simulink model "bloques_PMSM_v2"  (R2020b)
settings: Solver=VariableStepAuto  StartTime=0.0  StopTime=10.0  RelTol=1e-3
settings Model: Creator=JJVS  LastModifiedBy=jacob

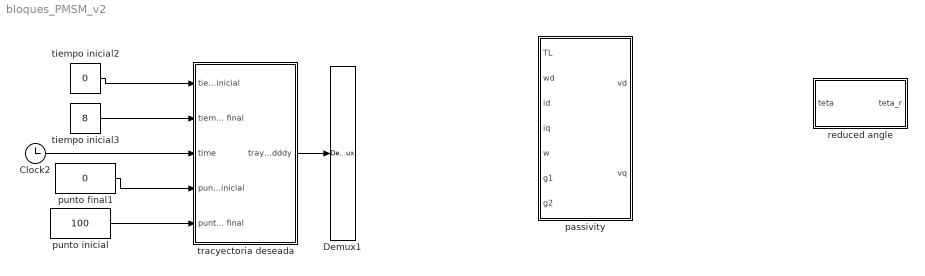
== system bloques_PMSM_v2 ==
  Clock2 : Clock
  Demux1 : Demux  Outputs=5
      settings: DisplayOption=none
  passivity : MATLAB Function  TreatAsAtomicUnit=on
  punto final1 : Constant  Value=0
  punto inicial : Constant  Value=100
  reduced angle : MATLAB Function  TreatAsAtomicUnit=on
  tiempo inicial2 : Constant  Value=0
  tiempo inicial3 : Constant  Value=8
  tracyectoria deseada : Subsystem
  wires:
  tiempo inicial2/1 -> tracyectoria deseada/1(tiempo inicial)
  tiempo inicial3/1 -> tracyectoria deseada/2(tiempo final)
  tracyectoria deseada/1(trayectoria y - ddddy) -> Demux1/1
  Clock2/1 -> tracyectoria deseada/3(time)
  punto inicial/1 -> tracyectoria deseada/5(punto final)
  punto final1/1 -> tracyectoria deseada/4(punto inicial)

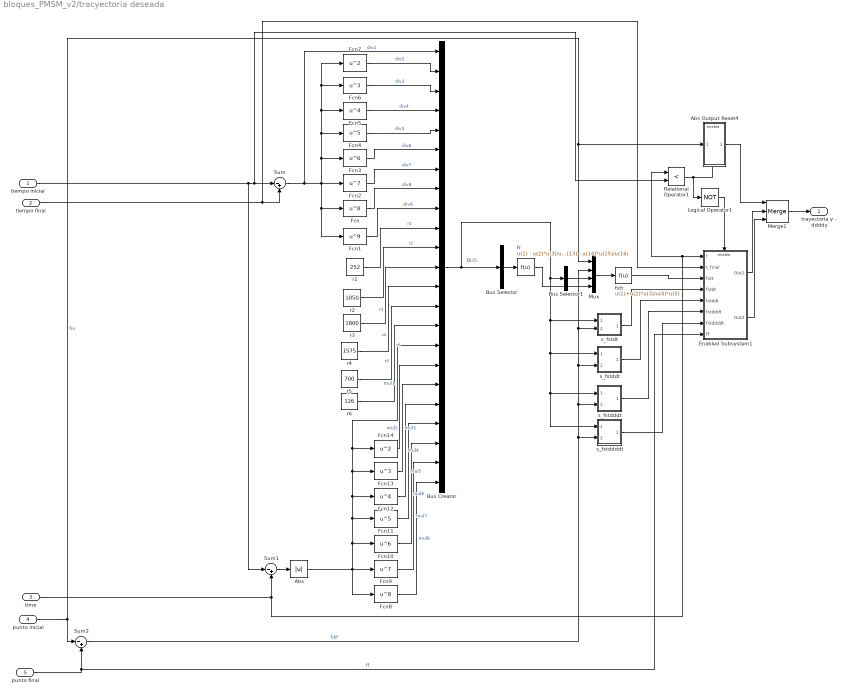
== system bloques_PMSM_v2/tracyectoria deseada ==
  note: BUS
  tiempo inicial : Inport
  tiempo final : Inport  Port=2
  time : Inport  Port=3
  punto inicial : Inport  Port=4
  punto final : Inport  Port=5
  Abs : Abs  SaturateOnIntegerOverflow=on
  Abs Output Reset4 : Subsystem  TreatAsAtomicUnit=on
  Bus Creator : BusCreator  Inputs=23
  Bus Selector : BusSelector  OutputSignals=r1,r2,mul1,div1,r3,mul2,div2,r4,mul3,div3,r5,mul4,div4,r6,mul5,div5  OutputAsBus=on
  Bus Selector1 : BusSelector  OutputSignals=mul5,div5  OutputAsBus=on
  Enabled Subsystem1 : Subsystem  TreatAsAtomicUnit=on
  Fcn : Fcn  Expr=u^8
  Fcn1 : Fcn  Expr=u^9
  Fcn10 : Fcn  Expr=u^6
  Fcn11 : Fcn  Expr=u^5
  Fcn12 : Fcn  Expr=u^4
  Fcn13 : Fcn  Expr=u^3
  Fcn14 : Fcn  Expr=u^2
  Fcn2 : Fcn  Expr=u^7
  Fcn3 : Fcn  Expr=u^6
  Fcn4 : Fcn  Expr=u^5
  Fcn5 : Fcn  Expr=u^4
  Fcn6 : Fcn  Expr=u^3
  Fcn7 : Fcn  Expr=u^2
  Fcn8 : Fcn  Expr=u^8
  Fcn9 : Fcn  Expr=u^7
  Logical Operator1 : Logic  Operator=NOT  AllPortsSameDT=off
  Merge1 : Merge  Inputs=3
  Mux : Mux
  Relational Operator1 : RelationalOperator  Operator=<  RndMeth=Nearest
  Sum : Sum  Inputs=|-+  SaturateOnIntegerOverflow=on
  Sum1 : Sum  Inputs=|-+  SaturateOnIntegerOverflow=on
  Sum2 : Sum  Inputs=|-+  SaturateOnIntegerOverflow=on
  fr : Fcn  Expr=u(1) - u(2)*u(3)/u(4)+u(5)*u(6)/u(7) - u(8)*u(9)/u(10) + u(11)*u(12)/u(13) - u(14)*u(15)/u(16)
  fstt : Fcn  Expr=u(1)+u(2)*u(3)/u(4)*u(5)
  r1 : Constant  Value=252
  r2 : Constant  Value=1050
  r3 : Constant  Value=1800
  r4 : Constant  Value=1575
  r5 : Constant  Value=700
  r6 : Constant  Value=126
  s_fstddddt : Subsystem
  s_fstdddt : Subsystem
  s_fstddt : Subsystem
  s_fstdt : Subsystem
  trayectoria y - ddddy : Outport  VectorParamsAs1DForOutWhenUnconnected=off
  wires:
  punto inicial/1 -> Mux/1, Abs Output Reset4/1(In1), Sum2/1  "fin"
  Bus Selector/1 -> fr/1
  Bus Selector1/1 -> Mux/3
  fr/1 -> Mux/4
  Mux/1 -> fstt/1
  punto final/1 -> Sum2/2, Enabled Subsystem1/8(ff)  "ff"
  tiempo inicial/1 -> Sum1/1, Sum/1, Relational Operator1/2
  Sum1/1 -> Abs/1
  Sum/1 -> Fcn2/1, Fcn3/1, Fcn4/1, Fcn5/1, Fcn6/1, Fcn7/1, Fcn/1, Fcn1/1, Bus Creator/1  "div1"
  Abs/1 -> Fcn13/1, Fcn14/1, Bus Creator/16, Fcn12/1, Fcn11/1, Fcn10/1, Fcn9/1, Fcn8/1  "mul1"
  Fcn7/1 -> Bus Creator/2  "div2"
  Fcn6/1 -> Bus Creator/3  "div3"
  Fcn5/1 -> Bus Creator/4  "div4"
  Fcn4/1 -> Bus Creator/5  "div5"
  Fcn3/1 -> Bus Creator/6  "div6"
  Fcn/1 -> Bus Creator/8  "div8"
  Fcn2/1 -> Bus Creator/7  "div7"
  Fcn1/1 -> Bus Creator/9  "div9"
  r1/1 -> Bus Creator/10  "r1"
  r2/1 -> Bus Creator/11  "r2"
  r3/1 -> Bus Creator/12  "r3"
  r4/1 -> Bus Creator/13  "r4"
  r5/1 -> Bus Creator/14  "r5"
  r6/1 -> Bus Creator/15  "r6"
  Fcn14/1 -> Bus Creator/17  "mul2"
  Fcn13/1 -> Bus Creator/18  "mul3"
  Fcn12/1 -> Bus Creator/19  "mul4"
  Fcn11/1 -> Bus Creator/20  "mul5"
  Fcn10/1 -> Bus Creator/21  "mul6"
  Fcn9/1 -> Bus Creator/22  "mul7"
  Fcn8/1 -> Bus Creator/23  "mul8"
  tiempo final/1 -> Sum/2, Enabled Subsystem1/2(t_final)
  time/1 -> Sum1/2, Enabled Subsystem1/1(t), Relational Operator1/1
  Merge1/1 -> trayectoria y - ddddy/1
  Bus Creator/1 -> Bus Selector1/1, s_fstdt/1(In1), s_fstddt/1(In1), s_fstdddt/1(In1), s_fstddddt/1(In1), Bus Selector/1
  Sum2/1 -> Mux/2, s_fstdt/2(In2), s_fstddt/2(In2), s_fstdddt/2(In2), s_fstddddt/2(In2)  "fdif"
  Relational Operator1/1 -> Abs Output Reset4/Enable, Logical Operator1/1
  Logical Operator1/1 -> Enabled Subsystem1/Enable
  Enabled Subsystem1/1(Out1) -> Merge1/2
  Abs Output Reset4/1(Out) -> Merge1/1
  fstt/1 -> Enabled Subsystem1/3(fstt)
  s_fstdt/1(fstdt) -> Enabled Subsystem1/4(fstdt)
  s_fstddt/1(fstddt) -> Enabled Subsystem1/5(fstddt)
  s_fstdddt/1(fstdddt) -> Enabled Subsystem1/6(fstdddt)
  s_fstddddt/1(fstddddt) -> Enabled Subsystem1/7(fstddddt)
  Enabled Subsystem1/2(Out2) -> Merge1/3

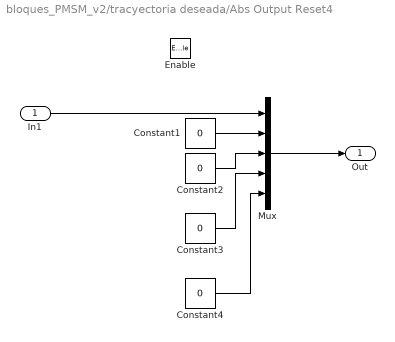
== system bloques_PMSM_v2/tracyectoria deseada/Abs Output Reset4 ==
  In1 : Inport  PortDimensions=1
  Enable : EnablePort
  Constant{1..4} (4 alike) : Constant  Value=0
  Mux : Mux  Inputs=5
  Out : Outport  InitialOutput=0  VectorParamsAs1DForOutWhenUnconnected=off
  wires:
  Mux/1 -> Out/1
  In1/1 -> Mux/1
  Constant1/1 -> Mux/2
  Constant2/1 -> Mux/3
  Constant3/1 -> Mux/4
  Constant4/1 -> Mux/5

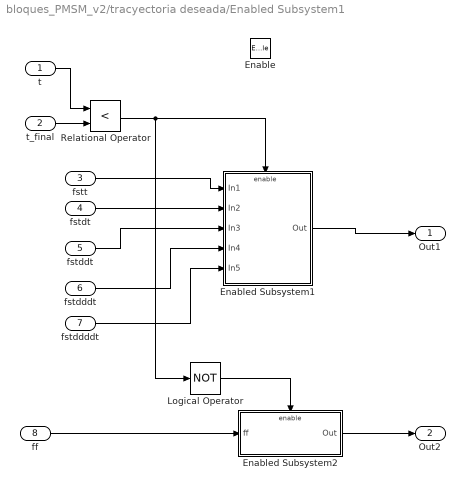
== system bloques_PMSM_v2/tracyectoria deseada/Enabled Subsystem1 ==
  t : Inport  PortDimensions=1
  t_final : Inport  Port=2  PortDimensions=1
  fstt : Inport  Port=3  PortDimensions=1
  fstdt : Inport  Port=4  PortDimensions=1
  fstddt : Inport  Port=5  PortDimensions=1
  fstdddt : Inport  Port=6  PortDimensions=1
  fstddddt : Inport  Port=7  PortDimensions=1
  ff : Inport  Port=8  PortDimensions=1
  Enable : EnablePort
  Enabled Subsystem1 : Subsystem  TreatAsAtomicUnit=on
  Enabled Subsystem2 : Subsystem  TreatAsAtomicUnit=on
  Logical Operator : Logic  Operator=NOT  AllPortsSameDT=off
  Relational Operator : RelationalOperator  Operator=<  RndMeth=Nearest
  Out1 : Outport  VectorParamsAs1DForOutWhenUnconnected=off
  Out2 : Outport  Port=2  VectorParamsAs1DForOutWhenUnconnected=off
  wires:
  Logical Operator/1 -> Enabled Subsystem2/Enable
  Relational Operator/1 -> Logical Operator/1, Enabled Subsystem1/Enable
  t/1 -> Relational Operator/1
  ff/1 -> Enabled Subsystem2/1(ff)
  fstt/1 -> Enabled Subsystem1/1(In1)
  fstdt/1 -> Enabled Subsystem1/2(In2)
  fstddt/1 -> Enabled Subsystem1/3(In3)
  fstdddt/1 -> Enabled Subsystem1/4(In4)
  fstddddt/1 -> Enabled Subsystem1/5(In5)
  t_final/1 -> Relational Operator/2
  Enabled Subsystem1/1(Out) -> Out1/1
  Enabled Subsystem2/1(Out) -> Out2/1

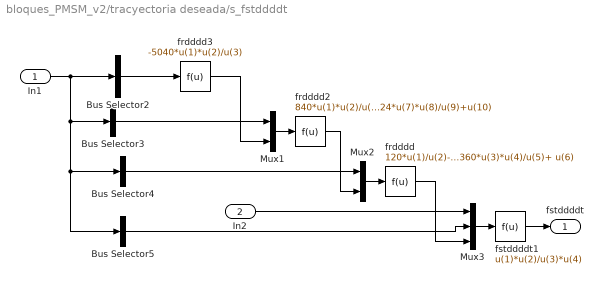
== system bloques_PMSM_v2/tracyectoria deseada/s_fstddddt ==
  In1 : Inport  PortDimensions=23
  In2 : Inport  Port=2  PortDimensions=1
  Bus Selector2 : BusSelector  OutputSignals=r6,mul5,div9  OutputAsBus=on
  Bus Selector3 : BusSelector  OutputSignals=r3,mul2,div6,r4,mul3,div7,r5,mul4,div8  OutputAsBus=on
  Bus Selector4 : BusSelector  OutputSignals=r1,div4,r2,mul1,div5  OutputAsBus=on
  Bus Selector5 : BusSelector  OutputSignals=mul1,div1  OutputAsBus=on
  Mux1 : Mux  Inputs=2
  Mux2 : Mux  Inputs=2
  Mux3 : Mux  Inputs=3
  frdddd : Fcn  Expr=120*u(1)/u(2)-360*u(3)*u(4)/u(5)+ u(6)
  frdddd2 : Fcn  Expr=840*u(1)*u(2)/u(3)-1680*u(4)*u(5)/u(6)+3024*u(7)*u(8)/u(9)+u(10)
  frdddd3 : Fcn  Expr=-5040*u(1)*u(2)/u(3)
  fstddddt1 : Fcn  Expr=u(1)*u(2)/u(3)*u(4)
  fstddddt : Outport  VectorParamsAs1DForOutWhenUnconnected=off
  wires:
  Bus Selector2/1 -> frdddd3/1
  Mux1/1 -> frdddd2/1
  frdddd3/1 -> Mux1/2
  Bus Selector3/1 -> Mux1/1
  Mux2/1 -> frdddd/1
  frdddd2/1 -> Mux2/2
  Bus Selector4/1 -> Mux2/1
  Mux3/1 -> fstddddt1/1
  frdddd/1 -> Mux3/3
  Bus Selector5/1 -> Mux3/2
  In1/1 -> Bus Selector2/1, Bus Selector3/1, Bus Selector4/1, Bus Selector5/1
  In2/1 -> Mux3/1
  fstddddt1/1 -> fstddddt/1

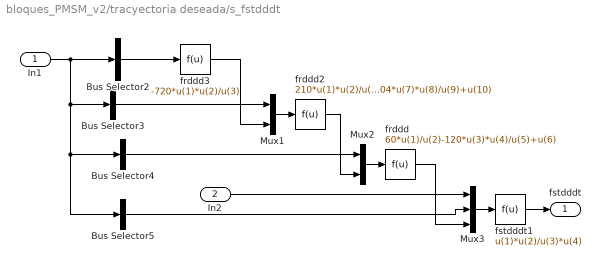
== system bloques_PMSM_v2/tracyectoria deseada/s_fstdddt ==
  In1 : Inport  PortDimensions=23
  In2 : Inport  Port=2  PortDimensions=1
  Bus Selector2 : BusSelector  OutputSignals=r6,mul5,div8  OutputAsBus=on
  Bus Selector3 : BusSelector  OutputSignals=r3,mul2,div5,r4,mul3,div6,r5,mul4,div7  OutputAsBus=on
  Bus Selector4 : BusSelector  OutputSignals=r1,div3,r2,mul1,div4  OutputAsBus=on
  Bus Selector5 : BusSelector  OutputSignals=mul2,div2  OutputAsBus=on
  Mux1 : Mux  Inputs=2
  Mux2 : Mux  Inputs=2
  Mux3 : Mux  Inputs=3
  frddd : Fcn  Expr=60*u(1)/u(2)-120*u(3)*u(4)/u(5)+u(6)
  frddd2 : Fcn  Expr=210*u(1)*u(2)/u(3)-336*u(4)*u(5)/u(6)+504*u(7)*u(8)/u(9)+u(10)
  frddd3 : Fcn  Expr=-720*u(1)*u(2)/u(3)
  fstdddt1 : Fcn  Expr=u(1)*u(2)/u(3)*u(4)
  fstdddt : Outport  VectorParamsAs1DForOutWhenUnconnected=off
  wires:
  fstdddt1/1 -> fstdddt/1
  In2/1 -> Mux3/1
  In1/1 -> Bus Selector5/1, Bus Selector4/1, Bus Selector3/1, Bus Selector2/1
  Bus Selector5/1 -> Mux3/2
  frddd/1 -> Mux3/3
  Mux3/1 -> fstdddt1/1
  Bus Selector4/1 -> Mux2/1
  frddd2/1 -> Mux2/2
  Mux2/1 -> frddd/1
  Bus Selector3/1 -> Mux1/1
  frddd3/1 -> Mux1/2
  Mux1/1 -> frddd2/1
  Bus Selector2/1 -> frddd3/1

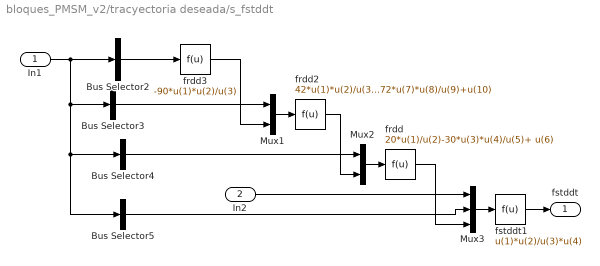
== system bloques_PMSM_v2/tracyectoria deseada/s_fstddt ==
  In1 : Inport  PortDimensions=23
  In2 : Inport  Port=2  PortDimensions=1
  Bus Selector2 : BusSelector  OutputSignals=r6,mul5,div7  OutputAsBus=on
  Bus Selector3 : BusSelector  OutputSignals=r3,mul2,div4,r4,mul3,div5,r5,mul4,div6  OutputAsBus=on
  Bus Selector4 : BusSelector  OutputSignals=r1,div2,r2,mul1,div3  OutputAsBus=on
  Bus Selector5 : BusSelector  OutputSignals=mul3,div3  OutputAsBus=on
  Mux1 : Mux  Inputs=2
  Mux2 : Mux  Inputs=2
  Mux3 : Mux  Inputs=3
  frdd : Fcn  Expr=20*u(1)/u(2)-30*u(3)*u(4)/u(5)+ u(6)
  frdd2 : Fcn  Expr=42*u(1)*u(2)/u(3)-56*u(4)*u(5)/u(6)+72*u(7)*u(8)/u(9)+u(10)
  frdd3 : Fcn  Expr=-90*u(1)*u(2)/u(3)
  fstddt1 : Fcn  Expr=u(1)*u(2)/u(3)*u(4)
  fstddt : Outport  VectorParamsAs1DForOutWhenUnconnected=off
  wires:
  Bus Selector2/1 -> frdd3/1
  Mux1/1 -> frdd2/1
  frdd3/1 -> Mux1/2
  Bus Selector3/1 -> Mux1/1
  Mux2/1 -> frdd/1
  frdd2/1 -> Mux2/2
  Bus Selector4/1 -> Mux2/1
  Mux3/1 -> fstddt1/1
  frdd/1 -> Mux3/3
  Bus Selector5/1 -> Mux3/2
  In1/1 -> Bus Selector2/1, Bus Selector3/1, Bus Selector4/1, Bus Selector5/1
  In2/1 -> Mux3/1
  fstddt1/1 -> fstddt/1

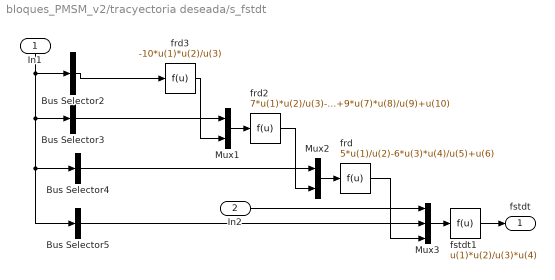
== system bloques_PMSM_v2/tracyectoria deseada/s_fstdt ==
  In1 : Inport  PortDimensions=23
  In2 : Inport  Port=2  PortDimensions=1
  Bus Selector2 : BusSelector  OutputSignals=r6,mul5,div6  OutputAsBus=on
  Bus Selector3 : BusSelector  OutputSignals=r3,mul2,div3,r4,mul3,div4,r5,mul4,div5  OutputAsBus=on
  Bus Selector4 : BusSelector  OutputSignals=r1,div1,r2,mul1,div2  OutputAsBus=on
  Bus Selector5 : BusSelector  OutputSignals=mul4,div4  OutputAsBus=on
  Mux1 : Mux  Inputs=2
  Mux2 : Mux  Inputs=2
  Mux3 : Mux  Inputs=3
  frd : Fcn  Expr=5*u(1)/u(2)-6*u(3)*u(4)/u(5)+u(6)
  frd2 : Fcn  Expr=7*u(1)*u(2)/u(3)-8*u(4)*u(5)/u(6)+9*u(7)*u(8)/u(9)+u(10)
  frd3 : Fcn  Expr=-10*u(1)*u(2)/u(3)
  fstdt1 : Fcn  Expr=u(1)*u(2)/u(3)*u(4)
  fstdt : Outport  VectorParamsAs1DForOutWhenUnconnected=off
  wires:
  Bus Selector2/1 -> frd3/1
  Mux1/1 -> frd2/1
  frd3/1 -> Mux1/2
  Bus Selector3/1 -> Mux1/1
  Mux2/1 -> frd/1
  frd2/1 -> Mux2/2
  Bus Selector4/1 -> Mux2/1
  Mux3/1 -> fstdt1/1
  frd/1 -> Mux3/3
  Bus Selector5/1 -> Mux3/2
  In1/1 -> Bus Selector2/1, Bus Selector3/1, Bus Selector4/1, Bus Selector5/1
  In2/1 -> Mux3/1
  fstdt1/1 -> fstdt/1

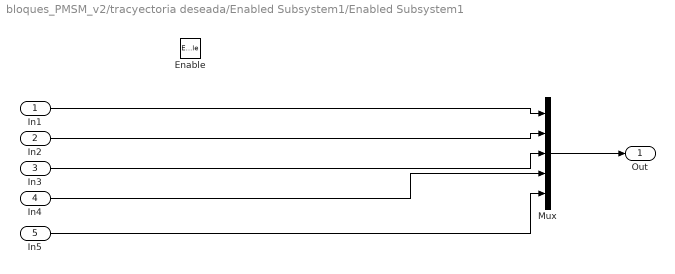
== system bloques_PMSM_v2/tracyectoria deseada/Enabled Subsystem1/Enabled Subsystem1 ==
  In1 : Inport  PortDimensions=1
  In2 : Inport  Port=2  PortDimensions=1
  In3 : Inport  Port=3  PortDimensions=1
  In4 : Inport  Port=4  PortDimensions=1
  In5 : Inport  Port=5  PortDimensions=1
  Enable : EnablePort
  Mux : Mux  Inputs=5
  Out : Outport  InitialOutput=0  VectorParamsAs1DForOutWhenUnconnected=off
  wires:
  Mux/1 -> Out/1
  In1/1 -> Mux/1
  In2/1 -> Mux/2
  In3/1 -> Mux/3
  In4/1 -> Mux/4
  In5/1 -> Mux/5

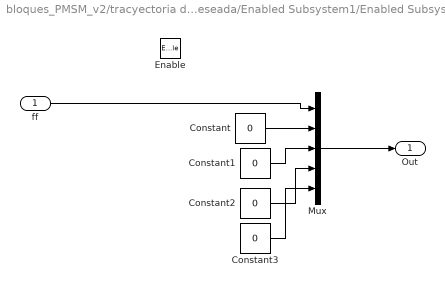
== system bloques_PMSM_v2/tracyectoria deseada/Enabled Subsystem1/Enabled Subsystem2 ==
  ff : Inport  PortDimensions=1
  Enable : EnablePort
  Constant{,1..3} (4 alike) : Constant  Value=0
  Mux : Mux  Inputs=5
  Out : Outport  InitialOutput=0  VectorParamsAs1DForOutWhenUnconnected=off
  wires:
  ff/1 -> Mux/1
  Mux/1 -> Out/1
  Constant3/1 -> Mux/5
  Constant2/1 -> Mux/4
  Constant1/1 -> Mux/3
  Constant/1 -> Mux/2

== matlab function bloques_PMSM_v2/reduced angle ==
  data: teta input; teta_r output
function teta_r = fcn(teta)

if (abs(teta)<2*pi)
    teta_r=abs(teta);
else
   aux1=abs(teta)/(2*pi);
   aux2=aux1-floor(aux1);
   teta_r=aux2*2*pi;
end

== matlab function bloques_PMSM_v2/passivity ==
  data: TL input; vd output; wd input; id input; iq input; w input; vq output; g1 input; g2 input
function [vd, vq]= fcn(TL, wd, id, iq, w, g1, g2)

Rs=1.6;
R=1.6;
Lq=6.635e-3;
Ld=6.635e-3;
L=Lq;
P=2;
J=0.182e-3;
Tau=2.09;
B=J/Tau;
%B=8.7E-5;
PhiPM=0.215;
%PhiPM=0.21309;
Km=P*PhiPM;

iqa=2/(3*Km)*(TL+B*wd);
vd=-P*L*w*iqa-g1*id;
vq=Km*wd+R*iqa-g2*(iq-iqa)
